simulink model "relative_logical_operation"  (R2020a)
settings: Solver=VariableStepAuto  StartTime=0.0  StopTime=10.0  RelTol=1e-3
settings Model: Creator=11973  LastModifiedBy=11973

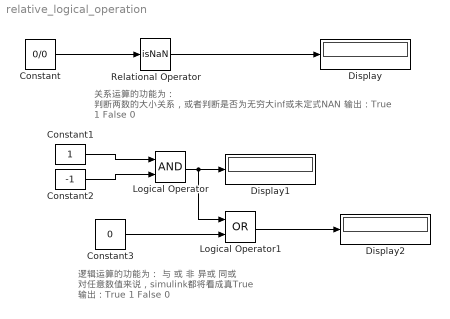
== system relative_logical_operation ==
  note: 关系运算的功能为：
      | 判断两数的大小关系，或者判断是否为无穷大inf或未定式NAN
      | 输出：True 1 False 0
  note: 逻辑运算的功能为：
      | 与 或 非 异或 同或
      | 对任意数值来说，simulink都将看成真True
      | 输出：True 1 False 0
  Constant : Constant  Value=0/0
  Constant1 : Constant
  Constant2 : Constant  Value=-1
  Constant3 : Constant  Value=0
  Display : Display
  Display1 : Display
  Display2 : Display
  Logical Operator : Logic  AllPortsSameDT=off  OutDataTypeStr=boolean
  Logical Operator1 : Logic  Operator=OR  AllPortsSameDT=off  OutDataTypeStr=boolean
  Relational Operator : RelationalOperator  Operator=isNaN  OutDataTypeStr=boolean  RndMeth=Simplest
  wires:
  Constant/1 -> Relational Operator/1
  Relational Operator/1 -> Display/1
  Constant1/1 -> Logical Operator/1
  Constant2/1 -> Logical Operator/2
  Logical Operator/1 -> Logical Operator1/1, Display1/1
  Constant3/1 -> Logical Operator1/2
  Logical Operator1/1 -> Display2/1
